simulink library "library"  (R2020a)
settings: Solver=VariableStepAuto  StartTime=0.0  StopTime=10.0  RelTol=1e-3
values from neighbouring files (symbols this model uses):
  height = 1080    [setup.m]    (also in setupSystem.m = heightName(nameIdx))
  nRho = maxRho*2    [setup.m]    (also in setupSystem.m)
  theta = (0:dTheta:180-dTheta)    [ARLHT.m]    (also in setup.m = (0:1:179); setupSystem.m = (0:1:179))
  width = 1920    [setup.m]    (also in setupSystem.m = widthName(nameIdx))
libraries: simulink x135, hdlsllib x83, $bdroot x15
(part 3 of 3)

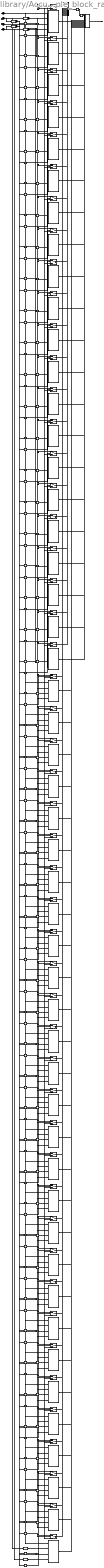
== system library/Accumulator Circuit/Accumulator Memory/Accumulator Memory/simple_block_ram ==
  wr_data : Inport
  wr_addr : Inport  Port=2
  wr_en : Inport  Port=3
  rd_addr : Inport  Port=4
  and_{0..48} (49 alike) : Logic  AllPortsSameDT=off  OutDataTypeStr=boolean
  bitwise_or : simulink/Logic and Bit Operations/Bitwise Operator  logicop=OR  UseBitMask=off  BitMask=bin2dec('11011001')  BitMaskRealWorld=Stored Integer
  constant_0 : Constant  Value=0  OutDataTypeStr=fixdt(0, 49, 0)  SampleTime=-1
  constant_1 : Constant  OutDataTypeStr=fixdt(0, 49, 0)  SampleTime=-1
  constant_10 : Constant  Value=10  OutDataTypeStr=fixdt(0, 49, 0)  SampleTime=-1
  constant_11 : Constant  Value=11  OutDataTypeStr=fixdt(0, 49, 0)  SampleTime=-1
  constant_12 : Constant  Value=12  OutDataTypeStr=fixdt(0, 49, 0)  SampleTime=-1
  constant_13 : Constant  Value=13  OutDataTypeStr=fixdt(0, 49, 0)  SampleTime=-1
  constant_14 : Constant  Value=14  OutDataTypeStr=fixdt(0, 49, 0)  SampleTime=-1
  constant_15 : Constant  Value=15  OutDataTypeStr=fixdt(0, 49, 0)  SampleTime=-1
  constant_16 : Constant  Value=16  OutDataTypeStr=fixdt(0, 49, 0)  SampleTime=-1
  constant_17 : Constant  Value=17  OutDataTypeStr=fixdt(0, 49, 0)  SampleTime=-1
  constant_18 : Constant  Value=18  OutDataTypeStr=fixdt(0, 49, 0)  SampleTime=-1
  constant_19 : Constant  Value=19  OutDataTypeStr=fixdt(0, 49, 0)  SampleTime=-1
  constant_2 : Constant  Value=2  OutDataTypeStr=fixdt(0, 49, 0)  SampleTime=-1
  constant_20 : Constant  Value=20  OutDataTypeStr=fixdt(0, 49, 0)  SampleTime=-1
  constant_21 : Constant  Value=21  OutDataTypeStr=fixdt(0, 49, 0)  SampleTime=-1
  constant_22 : Constant  Value=22  OutDataTypeStr=fixdt(0, 49, 0)  SampleTime=-1
  constant_23 : Constant  Value=23  OutDataTypeStr=fixdt(0, 49, 0)  SampleTime=-1
  constant_24 : Constant  Value=24  OutDataTypeStr=fixdt(0, 49, 0)  SampleTime=-1
  constant_25 : Constant  Value=25  OutDataTypeStr=fixdt(0, 49, 0)  SampleTime=-1
  constant_26 : Constant  Value=26  OutDataTypeStr=fixdt(0, 49, 0)  SampleTime=-1
  constant_27 : Constant  Value=27  OutDataTypeStr=fixdt(0, 49, 0)  SampleTime=-1
  constant_28 : Constant  Value=28  OutDataTypeStr=fixdt(0, 49, 0)  SampleTime=-1
  constant_29 : Constant  Value=29  OutDataTypeStr=fixdt(0, 49, 0)  SampleTime=-1
  constant_3 : Constant  Value=3  OutDataTypeStr=fixdt(0, 49, 0)  SampleTime=-1
  constant_30 : Constant  Value=30  OutDataTypeStr=fixdt(0, 49, 0)  SampleTime=-1
  constant_31 : Constant  Value=31  OutDataTypeStr=fixdt(0, 49, 0)  SampleTime=-1
  constant_32 : Constant  Value=32  OutDataTypeStr=fixdt(0, 49, 0)  SampleTime=-1
  constant_33 : Constant  Value=33  OutDataTypeStr=fixdt(0, 49, 0)  SampleTime=-1
  constant_34 : Constant  Value=34  OutDataTypeStr=fixdt(0, 49, 0)  SampleTime=-1
  constant_35 : Constant  Value=35  OutDataTypeStr=fixdt(0, 49, 0)  SampleTime=-1
  constant_36 : Constant  Value=36  OutDataTypeStr=fixdt(0, 49, 0)  SampleTime=-1
  constant_37 : Constant  Value=37  OutDataTypeStr=fixdt(0, 49, 0)  SampleTime=-1
  constant_38 : Constant  Value=38  OutDataTypeStr=fixdt(0, 49, 0)  SampleTime=-1
  constant_39 : Constant  Value=39  OutDataTypeStr=fixdt(0, 49, 0)  SampleTime=-1
  constant_4 : Constant  Value=4  OutDataTypeStr=fixdt(0, 49, 0)  SampleTime=-1
  constant_40 : Constant  Value=40  OutDataTypeStr=fixdt(0, 49, 0)  SampleTime=-1
  constant_41 : Constant  Value=41  OutDataTypeStr=fixdt(0, 49, 0)  SampleTime=-1
  constant_42 : Constant  Value=42  OutDataTypeStr=fixdt(0, 49, 0)  SampleTime=-1
  constant_43 : Constant  Value=43  OutDataTypeStr=fixdt(0, 49, 0)  SampleTime=-1
  constant_44 : Constant  Value=44  OutDataTypeStr=fixdt(0, 49, 0)  SampleTime=-1
  constant_45 : Constant  Value=45  OutDataTypeStr=fixdt(0, 49, 0)  SampleTime=-1
  constant_46 : Constant  Value=46  OutDataTypeStr=fixdt(0, 49, 0)  SampleTime=-1
  constant_47 : Constant  Value=47  OutDataTypeStr=fixdt(0, 49, 0)  SampleTime=-1
  constant_48 : Constant  Value=48  OutDataTypeStr=fixdt(0, 49, 0)  SampleTime=-1
  constant_5 : Constant  Value=5  OutDataTypeStr=fixdt(0, 49, 0)  SampleTime=-1
  constant_6 : Constant  Value=6  OutDataTypeStr=fixdt(0, 49, 0)  SampleTime=-1
  constant_7 : Constant  Value=7  OutDataTypeStr=fixdt(0, 49, 0)  SampleTime=-1
  constant_8 : Constant  Value=8  OutDataTypeStr=fixdt(0, 49, 0)  SampleTime=-1
  constant_9 : Constant  Value=9  OutDataTypeStr=fixdt(0, 49, 0)  SampleTime=-1
  delay : Delay  DelayLength=1
  multiport_switch : MultiPortSwitch  DataPortOrder=Zero-based contiguous  Inputs=49  zeroidx=on
  rd_address : hdlsllib/Logic and Bit Operations/Bit Slice  lidx=10  ridx=0
      settings: SourceProductBaseCode=SL
  rd_address_hr : hdlsllib/Logic and Bit Operations/Bit Slice  lidx=9  ridx=0
      settings: SourceProductBaseCode=SL
  rd_bitslice : hdlsllib/Logic and Bit Operations/Bit Slice  lidx=16  ridx=11
      settings: SourceProductBaseCode=SL
  rd_cmp2const_0 : simulink/Logic and Bit Operations/Compare To Constant  relop===  const=0  OutDataTypeStr=boolean
  rd_cmp2const_1 : simulink/Logic and Bit Operations/Compare To Constant  relop===  const=1  OutDataTypeStr=boolean
  rd_cmp2const_10 : simulink/Logic and Bit Operations/Compare To Constant  relop===  const=10  OutDataTypeStr=boolean
  rd_cmp2const_11 : simulink/Logic and Bit Operations/Compare To Constant  relop===  const=11  OutDataTypeStr=boolean
  rd_cmp2const_12 : simulink/Logic and Bit Operations/Compare To Constant  relop===  const=12  OutDataTypeStr=boolean
  rd_cmp2const_13 : simulink/Logic and Bit Operations/Compare To Constant  relop===  const=13  OutDataTypeStr=boolean
  rd_cmp2const_14 : simulink/Logic and Bit Operations/Compare To Constant  relop===  const=14  OutDataTypeStr=boolean
  rd_cmp2const_15 : simulink/Logic and Bit Operations/Compare To Constant  relop===  const=15  OutDataTypeStr=boolean
  rd_cmp2const_16 : simulink/Logic and Bit Operations/Compare To Constant  relop===  const=16  OutDataTypeStr=boolean
  rd_cmp2const_17 : simulink/Logic and Bit Operations/Compare To Constant  relop===  const=17  OutDataTypeStr=boolean
  rd_cmp2const_18 : simulink/Logic and Bit Operations/Compare To Constant  relop===  const=18  OutDataTypeStr=boolean
  rd_cmp2const_19 : simulink/Logic and Bit Operations/Compare To Constant  relop===  const=19  OutDataTypeStr=boolean
  rd_cmp2const_2 : simulink/Logic and Bit Operations/Compare To Constant  relop===  const=2  OutDataTypeStr=boolean
  rd_cmp2const_20 : simulink/Logic and Bit Operations/Compare To Constant  relop===  const=20  OutDataTypeStr=boolean
  rd_cmp2const_21 : simulink/Logic and Bit Operations/Compare To Constant  relop===  const=21  OutDataTypeStr=boolean
  rd_cmp2const_22 : simulink/Logic and Bit Operations/Compare To Constant  relop===  const=22  OutDataTypeStr=boolean
  rd_cmp2const_23 : simulink/Logic and Bit Operations/Compare To Constant  relop===  const=23  OutDataTypeStr=boolean
  rd_cmp2const_24 : simulink/Logic and Bit Operations/Compare To Constant  relop===  const=24  OutDataTypeStr=boolean
  rd_cmp2const_25 : simulink/Logic and Bit Operations/Compare To Constant  relop===  const=25  OutDataTypeStr=boolean
  rd_cmp2const_26 : simulink/Logic and Bit Operations/Compare To Constant  relop===  const=26  OutDataTypeStr=boolean
  rd_cmp2const_27 : simulink/Logic and Bit Operations/Compare To Constant  relop===  const=27  OutDataTypeStr=boolean
  rd_cmp2const_28 : simulink/Logic and Bit Operations/Compare To Constant  relop===  const=28  OutDataTypeStr=boolean
  rd_cmp2const_29 : simulink/Logic and Bit Operations/Compare To Constant  relop===  const=29  OutDataTypeStr=boolean
  rd_cmp2const_3 : simulink/Logic and Bit Operations/Compare To Constant  relop===  const=3  OutDataTypeStr=boolean
  rd_cmp2const_30 : simulink/Logic and Bit Operations/Compare To Constant  relop===  const=30  OutDataTypeStr=boolean
  rd_cmp2const_31 : simulink/Logic and Bit Operations/Compare To Constant  relop===  const=31  OutDataTypeStr=boolean
  rd_cmp2const_32 : simulink/Logic and Bit Operations/Compare To Constant  relop===  const=32  OutDataTypeStr=boolean
  rd_cmp2const_33 : simulink/Logic and Bit Operations/Compare To Constant  relop===  const=33  OutDataTypeStr=boolean
  rd_cmp2const_34 : simulink/Logic and Bit Operations/Compare To Constant  relop===  const=34  OutDataTypeStr=boolean
  rd_cmp2const_35 : simulink/Logic and Bit Operations/Compare To Constant  relop===  const=35  OutDataTypeStr=boolean
  rd_cmp2const_36 : simulink/Logic and Bit Operations/Compare To Constant  relop===  const=36  OutDataTypeStr=boolean
  rd_cmp2const_37 : simulink/Logic and Bit Operations/Compare To Constant  relop===  const=37  OutDataTypeStr=boolean
  rd_cmp2const_38 : simulink/Logic and Bit Operations/Compare To Constant  relop===  const=38  OutDataTypeStr=boolean
  rd_cmp2const_39 : simulink/Logic and Bit Operations/Compare To Constant  relop===  const=39  OutDataTypeStr=boolean
  rd_cmp2const_4 : simulink/Logic and Bit Operations/Compare To Constant  relop===  const=4  OutDataTypeStr=boolean
  rd_cmp2const_40 : simulink/Logic and Bit Operations/Compare To Constant  relop===  const=40  OutDataTypeStr=boolean
  rd_cmp2const_41 : simulink/Logic and Bit Operations/Compare To Constant  relop===  const=41  OutDataTypeStr=boolean
  rd_cmp2const_42 : simulink/Logic and Bit Operations/Compare To Constant  relop===  const=42  OutDataTypeStr=boolean
  rd_cmp2const_43 : simulink/Logic and Bit Operations/Compare To Constant  relop===  const=43  OutDataTypeStr=boolean
  rd_cmp2const_44 : simulink/Logic and Bit Operations/Compare To Constant  relop===  const=44  OutDataTypeStr=boolean
  rd_cmp2const_45 : simulink/Logic and Bit Operations/Compare To Constant  relop===  const=45  OutDataTypeStr=boolean
  rd_cmp2const_46 : simulink/Logic and Bit Operations/Compare To Constant  relop===  const=46  OutDataTypeStr=boolean
  rd_cmp2const_47 : simulink/Logic and Bit Operations/Compare To Constant  relop===  const=47  OutDataTypeStr=boolean
  rd_cmp2const_48 : simulink/Logic and Bit Operations/Compare To Constant  relop===  const=48  OutDataTypeStr=boolean
  rd_cmp2const_5 : simulink/Logic and Bit Operations/Compare To Constant  relop===  const=5  OutDataTypeStr=boolean
  rd_cmp2const_6 : simulink/Logic and Bit Operations/Compare To Constant  relop===  const=6  OutDataTypeStr=boolean
  rd_cmp2const_7 : simulink/Logic and Bit Operations/Compare To Constant  relop===  const=7  OutDataTypeStr=boolean
  rd_cmp2const_8 : simulink/Logic and Bit Operations/Compare To Constant  relop===  const=8  OutDataTypeStr=boolean
  rd_cmp2const_9 : simulink/Logic and Bit Operations/Compare To Constant  relop===  const=9  OutDataTypeStr=boolean
  simple_ram_{0..47} (48 alike) : hdlsllib/HDL RAMs/Simple Dual Port RAM  ram_size=11
      settings: SourceProductBaseCode=SL
  simple_ram_48 : hdlsllib/HDL RAMs/Simple Dual Port RAM  ram_size=10
      settings: SourceProductBaseCode=SL
  switch_{0..48} (49 alike) : Switch  Threshold=1
  vector_concatenate : Concatenate  NumInputs=49
  wr_address : hdlsllib/Logic and Bit Operations/Bit Slice  lidx=10  ridx=0
      settings: SourceProductBaseCode=SL
  wr_address_hr : hdlsllib/Logic and Bit Operations/Bit Slice  lidx=9  ridx=0
      settings: SourceProductBaseCode=SL
  wr_bitslice : hdlsllib/Logic and Bit Operations/Bit Slice  lidx=16  ridx=11
      settings: SourceProductBaseCode=SL
  wr_cmp2const_0 : simulink/Logic and Bit Operations/Compare To Constant  relop===  const=0  OutDataTypeStr=boolean
  wr_cmp2const_1 : simulink/Logic and Bit Operations/Compare To Constant  relop===  const=1  OutDataTypeStr=boolean
  wr_cmp2const_10 : simulink/Logic and Bit Operations/Compare To Constant  relop===  const=10  OutDataTypeStr=boolean
  wr_cmp2const_11 : simulink/Logic and Bit Operations/Compare To Constant  relop===  const=11  OutDataTypeStr=boolean
  wr_cmp2const_12 : simulink/Logic and Bit Operations/Compare To Constant  relop===  const=12  OutDataTypeStr=boolean
  wr_cmp2const_13 : simulink/Logic and Bit Operations/Compare To Constant  relop===  const=13  OutDataTypeStr=boolean
  wr_cmp2const_14 : simulink/Logic and Bit Operations/Compare To Constant  relop===  const=14  OutDataTypeStr=boolean
  wr_cmp2const_15 : simulink/Logic and Bit Operations/Compare To Constant  relop===  const=15  OutDataTypeStr=boolean
  wr_cmp2const_16 : simulink/Logic and Bit Operations/Compare To Constant  relop===  const=16  OutDataTypeStr=boolean
  wr_cmp2const_17 : simulink/Logic and Bit Operations/Compare To Constant  relop===  const=17  OutDataTypeStr=boolean
  wr_cmp2const_18 : simulink/Logic and Bit Operations/Compare To Constant  relop===  const=18  OutDataTypeStr=boolean
  wr_cmp2const_19 : simulink/Logic and Bit Operations/Compare To Constant  relop===  const=19  OutDataTypeStr=boolean
  wr_cmp2const_2 : simulink/Logic and Bit Operations/Compare To Constant  relop===  const=2  OutDataTypeStr=boolean
  wr_cmp2const_20 : simulink/Logic and Bit Operations/Compare To Constant  relop===  const=20  OutDataTypeStr=boolean
  wr_cmp2const_21 : simulink/Logic and Bit Operations/Compare To Constant  relop===  const=21  OutDataTypeStr=boolean
  wr_cmp2const_22 : simulink/Logic and Bit Operations/Compare To Constant  relop===  const=22  OutDataTypeStr=boolean
  wr_cmp2const_23 : simulink/Logic and Bit Operations/Compare To Constant  relop===  const=23  OutDataTypeStr=boolean
  wr_cmp2const_24 : simulink/Logic and Bit Operations/Compare To Constant  relop===  const=24  OutDataTypeStr=boolean
  wr_cmp2const_25 : simulink/Logic and Bit Operations/Compare To Constant  relop===  const=25  OutDataTypeStr=boolean
  wr_cmp2const_26 : simulink/Logic and Bit Operations/Compare To Constant  relop===  const=26  OutDataTypeStr=boolean
  wr_cmp2const_27 : simulink/Logic and Bit Operations/Compare To Constant  relop===  const=27  OutDataTypeStr=boolean
  wr_cmp2const_28 : simulink/Logic and Bit Operations/Compare To Constant  relop===  const=28  OutDataTypeStr=boolean
  wr_cmp2const_29 : simulink/Logic and Bit Operations/Compare To Constant  relop===  const=29  OutDataTypeStr=boolean
  wr_cmp2const_3 : simulink/Logic and Bit Operations/Compare To Constant  relop===  const=3  OutDataTypeStr=boolean
  wr_cmp2const_30 : simulink/Logic and Bit Operations/Compare To Constant  relop===  const=30  OutDataTypeStr=boolean
  wr_cmp2const_31 : simulink/Logic and Bit Operations/Compare To Constant  relop===  const=31  OutDataTypeStr=boolean
  wr_cmp2const_32 : simulink/Logic and Bit Operations/Compare To Constant  relop===  const=32  OutDataTypeStr=boolean
  wr_cmp2const_33 : simulink/Logic and Bit Operations/Compare To Constant  relop===  const=33  OutDataTypeStr=boolean
  wr_cmp2const_34 : simulink/Logic and Bit Operations/Compare To Constant  relop===  const=34  OutDataTypeStr=boolean
  wr_cmp2const_35 : simulink/Logic and Bit Operations/Compare To Constant  relop===  const=35  OutDataTypeStr=boolean
  wr_cmp2const_36 : simulink/Logic and Bit Operations/Compare To Constant  relop===  const=36  OutDataTypeStr=boolean
  wr_cmp2const_37 : simulink/Logic and Bit Operations/Compare To Constant  relop===  const=37  OutDataTypeStr=boolean
  wr_cmp2const_38 : simulink/Logic and Bit Operations/Compare To Constant  relop===  const=38  OutDataTypeStr=boolean
  wr_cmp2const_39 : simulink/Logic and Bit Operations/Compare To Constant  relop===  const=39  OutDataTypeStr=boolean
  wr_cmp2const_4 : simulink/Logic and Bit Operations/Compare To Constant  relop===  const=4  OutDataTypeStr=boolean
  wr_cmp2const_40 : simulink/Logic and Bit Operations/Compare To Constant  relop===  const=40  OutDataTypeStr=boolean
  wr_cmp2const_41 : simulink/Logic and Bit Operations/Compare To Constant  relop===  const=41  OutDataTypeStr=boolean
  wr_cmp2const_42 : simulink/Logic and Bit Operations/Compare To Constant  relop===  const=42  OutDataTypeStr=boolean
  wr_cmp2const_43 : simulink/Logic and Bit Operations/Compare To Constant  relop===  const=43  OutDataTypeStr=boolean
  wr_cmp2const_44 : simulink/Logic and Bit Operations/Compare To Constant  relop===  const=44  OutDataTypeStr=boolean
  wr_cmp2const_45 : simulink/Logic and Bit Operations/Compare To Constant  relop===  const=45  OutDataTypeStr=boolean
  wr_cmp2const_46 : simulink/Logic and Bit Operations/Compare To Constant  relop===  const=46  OutDataTypeStr=boolean
  wr_cmp2const_47 : simulink/Logic and Bit Operations/Compare To Constant  relop===  const=47  OutDataTypeStr=boolean
  wr_cmp2const_48 : simulink/Logic and Bit Operations/Compare To Constant  relop===  const=48  OutDataTypeStr=boolean
  wr_cmp2const_5 : simulink/Logic and Bit Operations/Compare To Constant  relop===  const=5  OutDataTypeStr=boolean
  wr_cmp2const_6 : simulink/Logic and Bit Operations/Compare To Constant  relop===  const=6  OutDataTypeStr=boolean
  wr_cmp2const_7 : simulink/Logic and Bit Operations/Compare To Constant  relop===  const=7  OutDataTypeStr=boolean
  wr_cmp2const_8 : simulink/Logic and Bit Operations/Compare To Constant  relop===  const=8  OutDataTypeStr=boolean
  wr_cmp2const_9 : simulink/Logic and Bit Operations/Compare To Constant  relop===  const=9  OutDataTypeStr=boolean
  zero : Constant  Value=0  OutDataTypeStr=fixdt(0, 49, 0)  SampleTime=-1
  rd_data : Outport
  wires:
  wr_data/1 -> simple_ram_0/1, simple_ram_1/1, simple_ram_2/1, simple_ram_3/1, simple_ram_4/1, simple_ram_5/1, simple_ram_6/1, simple_ram_7/1, simple_ram_8/1, simple_ram_9/1, simple_ram_10/1, simple_ram_11/1, simple_ram_12/1, simple_ram_13/1, simple_ram_14/1, simple_ram_15/1, simple_ram_16/1, simple_ram_17/1, simple_ram_18/1, simple_ram_19/1, simple_ram_20/1, simple_ram_21/1, simple_ram_22/1, simple_ram_23/1, simple_ram_24/1, simple_ram_25/1, simple_ram_26/1, simple_ram_27/1, simple_ram_28/1, simple_ram_29/1, simple_ram_30/1, simple_ram_31/1, simple_ram_32/1, simple_ram_33/1, simple_ram_34/1, simple_ram_35/1, simple_ram_36/1, simple_ram_37/1, simple_ram_38/1, simple_ram_39/1, simple_ram_40/1, simple_ram_41/1, simple_ram_42/1, simple_ram_43/1, simple_ram_44/1, simple_ram_45/1, simple_ram_46/1, simple_ram_47/1, simple_ram_48/1
  wr_address/1 -> simple_ram_0/2, simple_ram_1/2, simple_ram_2/2, simple_ram_3/2, simple_ram_4/2, simple_ram_5/2, simple_ram_6/2, simple_ram_7/2, simple_ram_8/2, simple_ram_9/2, simple_ram_10/2, simple_ram_11/2, simple_ram_12/2, simple_ram_13/2, simple_ram_14/2, simple_ram_15/2, simple_ram_16/2, simple_ram_17/2, simple_ram_18/2, simple_ram_19/2, simple_ram_20/2, simple_ram_21/2, simple_ram_22/2, simple_ram_23/2, simple_ram_24/2, simple_ram_25/2, simple_ram_26/2, simple_ram_27/2, simple_ram_28/2, simple_ram_29/2, simple_ram_30/2, simple_ram_31/2, simple_ram_32/2, simple_ram_33/2, simple_ram_34/2, simple_ram_35/2, simple_ram_36/2, simple_ram_37/2, simple_ram_38/2, simple_ram_39/2, simple_ram_40/2, simple_ram_41/2, simple_ram_42/2, simple_ram_43/2, simple_ram_44/2, simple_ram_45/2, simple_ram_46/2, simple_ram_47/2
  rd_address/1 -> simple_ram_0/4, simple_ram_1/4, simple_ram_2/4, simple_ram_3/4, simple_ram_4/4, simple_ram_5/4, simple_ram_6/4, simple_ram_7/4, simple_ram_8/4, simple_ram_9/4, simple_ram_10/4, simple_ram_11/4, simple_ram_12/4, simple_ram_13/4, simple_ram_14/4, simple_ram_15/4, simple_ram_16/4, simple_ram_17/4, simple_ram_18/4, simple_ram_19/4, simple_ram_20/4, simple_ram_21/4, simple_ram_22/4, simple_ram_23/4, simple_ram_24/4, simple_ram_25/4, simple_ram_26/4, simple_ram_27/4, simple_ram_28/4, simple_ram_29/4, simple_ram_30/4, simple_ram_31/4, simple_ram_32/4, simple_ram_33/4, simple_ram_34/4, simple_ram_35/4, simple_ram_36/4, simple_ram_37/4, simple_ram_38/4, simple_ram_39/4, simple_ram_40/4, simple_ram_41/4, simple_ram_42/4, simple_ram_43/4, simple_ram_44/4, simple_ram_45/4, simple_ram_46/4, simple_ram_47/4
  constant_0/1 -> switch_0/1
  zero/1 -> switch_0/3, switch_1/3, switch_2/3, switch_3/3, switch_4/3, switch_5/3, switch_6/3, switch_7/3, switch_8/3, switch_9/3, switch_10/3, switch_11/3, switch_12/3, switch_13/3, switch_14/3, switch_15/3, switch_16/3, switch_17/3, switch_18/3, switch_19/3, switch_20/3, switch_21/3, switch_22/3, switch_23/3, switch_24/3, switch_25/3, switch_26/3, switch_27/3, switch_28/3, switch_29/3, switch_30/3, switch_31/3, switch_32/3, switch_33/3, switch_34/3, switch_35/3, switch_36/3, switch_37/3, switch_38/3, switch_39/3, switch_40/3, switch_41/3, switch_42/3, switch_43/3, switch_44/3, switch_45/3, switch_46/3, switch_47/3, switch_48/3
  switch_0/1 -> vector_concatenate/1
  simple_ram_0/1 -> multiport_switch/2
  wr_bitslice/1 -> wr_cmp2const_0/1, wr_cmp2const_1/1, wr_cmp2const_2/1, wr_cmp2const_3/1, wr_cmp2const_4/1, wr_cmp2const_5/1, wr_cmp2const_6/1, wr_cmp2const_7/1, wr_cmp2const_8/1, wr_cmp2const_9/1, wr_cmp2const_10/1, wr_cmp2const_11/1, wr_cmp2const_12/1, wr_cmp2const_13/1, wr_cmp2const_14/1, wr_cmp2const_15/1, wr_cmp2const_16/1, wr_cmp2const_17/1, wr_cmp2const_18/1, wr_cmp2const_19/1, wr_cmp2const_20/1, wr_cmp2const_21/1, wr_cmp2const_22/1, wr_cmp2const_23/1, wr_cmp2const_24/1, wr_cmp2const_25/1, wr_cmp2const_26/1, wr_cmp2const_27/1, wr_cmp2const_28/1, wr_cmp2const_29/1, wr_cmp2const_30/1, wr_cmp2const_31/1, wr_cmp2const_32/1, wr_cmp2const_33/1, wr_cmp2const_34/1, wr_cmp2const_35/1, wr_cmp2const_36/1, wr_cmp2const_37/1, wr_cmp2const_38/1, wr_cmp2const_39/1, wr_cmp2const_40/1, wr_cmp2const_41/1, wr_cmp2const_42/1, wr_cmp2const_43/1, wr_cmp2const_44/1, wr_cmp2const_45/1, wr_cmp2const_46/1, wr_cmp2const_47/1, wr_cmp2const_48/1
  rd_bitslice/1 -> rd_cmp2const_0/1, rd_cmp2const_1/1, rd_cmp2const_2/1, rd_cmp2const_3/1, rd_cmp2const_4/1, rd_cmp2const_5/1, rd_cmp2const_6/1, rd_cmp2const_7/1, rd_cmp2const_8/1, rd_cmp2const_9/1, rd_cmp2const_10/1, rd_cmp2const_11/1, rd_cmp2const_12/1, rd_cmp2const_13/1, rd_cmp2const_14/1, rd_cmp2const_15/1, rd_cmp2const_16/1, rd_cmp2const_17/1, rd_cmp2const_18/1, rd_cmp2const_19/1, rd_cmp2const_20/1, rd_cmp2const_21/1, rd_cmp2const_22/1, rd_cmp2const_23/1, rd_cmp2const_24/1, rd_cmp2const_25/1, rd_cmp2const_26/1, rd_cmp2const_27/1, rd_cmp2const_28/1, rd_cmp2const_29/1, rd_cmp2const_30/1, rd_cmp2const_31/1, rd_cmp2const_32/1, rd_cmp2const_33/1, rd_cmp2const_34/1, rd_cmp2const_35/1, rd_cmp2const_36/1, rd_cmp2const_37/1, rd_cmp2const_38/1, rd_cmp2const_39/1, rd_cmp2const_40/1, rd_cmp2const_41/1, rd_cmp2const_42/1, rd_cmp2const_43/1, rd_cmp2const_44/1, rd_cmp2const_45/1, rd_cmp2const_46/1, rd_cmp2const_47/1, rd_cmp2const_48/1
  wr_en/1 -> and_0/2, and_1/2, and_2/2, and_3/2, and_4/2, and_5/2, and_6/2, and_7/2, and_8/2, and_9/2, and_10/2, and_11/2, and_12/2, and_13/2, and_14/2, and_15/2, and_16/2, and_17/2, and_18/2, and_19/2, and_20/2, and_21/2, and_22/2, and_23/2, and_24/2, and_25/2, and_26/2, and_27/2, and_28/2, and_29/2, and_30/2, and_31/2, and_32/2, and_33/2, and_34/2, and_35/2, and_36/2, and_37/2, and_38/2, and_39/2, and_40/2, and_41/2, and_42/2, and_43/2, and_44/2, and_45/2, and_46/2, and_47/2, and_48/2
  and_0/1 -> simple_ram_0/3
  wr_cmp2const_0/1 -> and_0/1
  rd_cmp2const_0/1 -> switch_0/2
  constant_1/1 -> switch_1/1
  switch_1/1 -> vector_concatenate/2
  simple_ram_1/1 -> multiport_switch/3
  and_1/1 -> simple_ram_1/3
  wr_cmp2const_1/1 -> and_1/1
  rd_cmp2const_1/1 -> switch_1/2
  constant_2/1 -> switch_2/1
  switch_2/1 -> vector_concatenate/3
  simple_ram_2/1 -> multiport_switch/4
  and_2/1 -> simple_ram_2/3
  wr_cmp2const_2/1 -> and_2/1
  rd_cmp2const_2/1 -> switch_2/2
  constant_3/1 -> switch_3/1
  switch_3/1 -> vector_concatenate/4
  simple_ram_3/1 -> multiport_switch/5
  and_3/1 -> simple_ram_3/3
  wr_cmp2const_3/1 -> and_3/1
  rd_cmp2const_3/1 -> switch_3/2
  constant_4/1 -> switch_4/1
  switch_4/1 -> vector_concatenate/5
  simple_ram_4/1 -> multiport_switch/6
  and_4/1 -> simple_ram_4/3
  wr_cmp2const_4/1 -> and_4/1
  rd_cmp2const_4/1 -> switch_4/2
  constant_5/1 -> switch_5/1
  switch_5/1 -> vector_concatenate/6
  simple_ram_5/1 -> multiport_switch/7
  and_5/1 -> simple_ram_5/3
  wr_cmp2const_5/1 -> and_5/1
  rd_cmp2const_5/1 -> switch_5/2
  constant_6/1 -> switch_6/1
  switch_6/1 -> vector_concatenate/7
  simple_ram_6/1 -> multiport_switch/8
  and_6/1 -> simple_ram_6/3
  wr_cmp2const_6/1 -> and_6/1
  rd_cmp2const_6/1 -> switch_6/2
  constant_7/1 -> switch_7/1
  switch_7/1 -> vector_concatenate/8
  simple_ram_7/1 -> multiport_switch/9
  and_7/1 -> simple_ram_7/3
  wr_cmp2const_7/1 -> and_7/1
  rd_cmp2const_7/1 -> switch_7/2
  constant_8/1 -> switch_8/1
  switch_8/1 -> vector_concatenate/9
  simple_ram_8/1 -> multiport_switch/10
  and_8/1 -> simple_ram_8/3
  wr_cmp2const_8/1 -> and_8/1
  rd_cmp2const_8/1 -> switch_8/2
  constant_9/1 -> switch_9/1
  switch_9/1 -> vector_concatenate/10
  simple_ram_9/1 -> multiport_switch/11
  and_9/1 -> simple_ram_9/3
  wr_cmp2const_9/1 -> and_9/1
  rd_cmp2const_9/1 -> switch_9/2
  constant_10/1 -> switch_10/1
  switch_10/1 -> vector_concatenate/11
  simple_ram_10/1 -> multiport_switch/12
  and_10/1 -> simple_ram_10/3
  wr_cmp2const_10/1 -> and_10/1
  rd_cmp2const_10/1 -> switch_10/2
  constant_11/1 -> switch_11/1
  switch_11/1 -> vector_concatenate/12
  simple_ram_11/1 -> multiport_switch/13
  and_11/1 -> simple_ram_11/3
  wr_cmp2const_11/1 -> and_11/1
  rd_cmp2const_11/1 -> switch_11/2
  constant_12/1 -> switch_12/1
  switch_12/1 -> vector_concatenate/13
  simple_ram_12/1 -> multiport_switch/14
  and_12/1 -> simple_ram_12/3
  wr_cmp2const_12/1 -> and_12/1
  rd_cmp2const_12/1 -> switch_12/2
  constant_13/1 -> switch_13/1
  switch_13/1 -> vector_concatenate/14
  simple_ram_13/1 -> multiport_switch/15
  and_13/1 -> simple_ram_13/3
  wr_cmp2const_13/1 -> and_13/1
  rd_cmp2const_13/1 -> switch_13/2
  constant_14/1 -> switch_14/1
  switch_14/1 -> vector_concatenate/15
  simple_ram_14/1 -> multiport_switch/16
  and_14/1 -> simple_ram_14/3
  wr_cmp2const_14/1 -> and_14/1
  rd_cmp2const_14/1 -> switch_14/2
  constant_15/1 -> switch_15/1
  switch_15/1 -> vector_concatenate/16
  simple_ram_15/1 -> multiport_switch/17
  and_15/1 -> simple_ram_15/3
  wr_cmp2const_15/1 -> and_15/1
  rd_cmp2const_15/1 -> switch_15/2
  constant_16/1 -> switch_16/1
  switch_16/1 -> vector_concatenate/17
  simple_ram_16/1 -> multiport_switch/18
  and_16/1 -> simple_ram_16/3
  wr_cmp2const_16/1 -> and_16/1
  rd_cmp2const_16/1 -> switch_16/2
  constant_17/1 -> switch_17/1
  switch_17/1 -> vector_concatenate/18
  simple_ram_17/1 -> multiport_switch/19
  and_17/1 -> simple_ram_17/3
  wr_cmp2const_17/1 -> and_17/1
  rd_cmp2const_17/1 -> switch_17/2
  constant_18/1 -> switch_18/1
  switch_18/1 -> vector_concatenate/19
  simple_ram_18/1 -> multiport_switch/20
  and_18/1 -> simple_ram_18/3
  wr_cmp2const_18/1 -> and_18/1
  rd_cmp2const_18/1 -> switch_18/2
  constant_19/1 -> switch_19/1
  switch_19/1 -> vector_concatenate/20
  simple_ram_19/1 -> multiport_switch/21
  and_19/1 -> simple_ram_19/3
  wr_cmp2const_19/1 -> and_19/1
  rd_cmp2const_19/1 -> switch_19/2
  constant_20/1 -> switch_20/1
  switch_20/1 -> vector_concatenate/21
  simple_ram_20/1 -> multiport_switch/22
  and_20/1 -> simple_ram_20/3
  wr_cmp2const_20/1 -> and_20/1
  rd_cmp2const_20/1 -> switch_20/2
  constant_21/1 -> switch_21/1
  switch_21/1 -> vector_concatenate/22
  simple_ram_21/1 -> multiport_switch/23
  and_21/1 -> simple_ram_21/3
  wr_cmp2const_21/1 -> and_21/1
  rd_cmp2const_21/1 -> switch_21/2
  constant_22/1 -> switch_22/1
  switch_22/1 -> vector_concatenate/23
  simple_ram_22/1 -> multiport_switch/24
  and_22/1 -> simple_ram_22/3
  wr_cmp2const_22/1 -> and_22/1
  rd_cmp2const_22/1 -> switch_22/2
  constant_23/1 -> switch_23/1
  switch_23/1 -> vector_concatenate/24
  simple_ram_23/1 -> multiport_switch/25
  and_23/1 -> simple_ram_23/3
  wr_cmp2const_23/1 -> and_23/1
  rd_cmp2const_23/1 -> switch_23/2
  constant_24/1 -> switch_24/1
  switch_24/1 -> vector_concatenate/25
  simple_ram_24/1 -> multiport_switch/26
  and_24/1 -> simple_ram_24/3
  wr_cmp2const_24/1 -> and_24/1
  rd_cmp2const_24/1 -> switch_24/2
  constant_25/1 -> switch_25/1
  switch_25/1 -> vector_concatenate/26
  simple_ram_25/1 -> multiport_switch/27
  and_25/1 -> simple_ram_25/3
  wr_cmp2const_25/1 -> and_25/1
  rd_cmp2const_25/1 -> switch_25/2
  constant_26/1 -> switch_26/1
  switch_26/1 -> vector_concatenate/27
  simple_ram_26/1 -> multiport_switch/28
  and_26/1 -> simple_ram_26/3
  wr_cmp2const_26/1 -> and_26/1
  rd_cmp2const_26/1 -> switch_26/2
  constant_27/1 -> switch_27/1
  switch_27/1 -> vector_concatenate/28
  simple_ram_27/1 -> multiport_switch/29
  and_27/1 -> simple_ram_27/3
  wr_cmp2const_27/1 -> and_27/1
  rd_cmp2const_27/1 -> switch_27/2
  constant_28/1 -> switch_28/1
  switch_28/1 -> vector_concatenate/29
  simple_ram_28/1 -> multiport_switch/30
  and_28/1 -> simple_ram_28/3
  wr_cmp2const_28/1 -> and_28/1
  rd_cmp2const_28/1 -> switch_28/2
  constant_29/1 -> switch_29/1
  switch_29/1 -> vector_concatenate/30
  simple_ram_29/1 -> multiport_switch/31
  and_29/1 -> simple_ram_29/3
  wr_cmp2const_29/1 -> and_29/1
  rd_cmp2const_29/1 -> switch_29/2
  constant_30/1 -> switch_30/1
  switch_30/1 -> vector_concatenate/31
  simple_ram_30/1 -> multiport_switch/32
  and_30/1 -> simple_ram_30/3
  wr_cmp2const_30/1 -> and_30/1
  rd_cmp2const_30/1 -> switch_30/2
  constant_31/1 -> switch_31/1
  switch_31/1 -> vector_concatenate/32
  simple_ram_31/1 -> multiport_switch/33
  and_31/1 -> simple_ram_31/3
  wr_cmp2const_31/1 -> and_31/1
  rd_cmp2const_31/1 -> switch_31/2
  constant_32/1 -> switch_32/1
  switch_32/1 -> vector_concatenate/33
  simple_ram_32/1 -> multiport_switch/34
  and_32/1 -> simple_ram_32/3
  wr_cmp2const_32/1 -> and_32/1
  rd_cmp2const_32/1 -> switch_32/2
  constant_33/1 -> switch_33/1
  switch_33/1 -> vector_concatenate/34
  simple_ram_33/1 -> multiport_switch/35
  and_33/1 -> simple_ram_33/3
  wr_cmp2const_33/1 -> and_33/1
  rd_cmp2const_33/1 -> switch_33/2
  constant_34/1 -> switch_34/1
  switch_34/1 -> vector_concatenate/35
  simple_ram_34/1 -> multiport_switch/36
  and_34/1 -> simple_ram_34/3
  wr_cmp2const_34/1 -> and_34/1
  rd_cmp2const_34/1 -> switch_34/2
  constant_35/1 -> switch_35/1
  switch_35/1 -> vector_concatenate/36
  simple_ram_35/1 -> multiport_switch/37
  and_35/1 -> simple_ram_35/3
  wr_cmp2const_35/1 -> and_35/1
  rd_cmp2const_35/1 -> switch_35/2
  constant_36/1 -> switch_36/1
  switch_36/1 -> vector_concatenate/37
  simple_ram_36/1 -> multiport_switch/38
  and_36/1 -> simple_ram_36/3
  wr_cmp2const_36/1 -> and_36/1
  rd_cmp2const_36/1 -> switch_36/2
  constant_37/1 -> switch_37/1
  switch_37/1 -> vector_concatenate/38
  simple_ram_37/1 -> multiport_switch/39
  and_37/1 -> simple_ram_37/3
  wr_cmp2const_37/1 -> and_37/1
  rd_cmp2const_37/1 -> switch_37/2
  constant_38/1 -> switch_38/1
  switch_38/1 -> vector_concatenate/39
  simple_ram_38/1 -> multiport_switch/40
  and_38/1 -> simple_ram_38/3
  wr_cmp2const_38/1 -> and_38/1
  rd_cmp2const_38/1 -> switch_38/2
  constant_39/1 -> switch_39/1
  switch_39/1 -> vector_concatenate/40
  simple_ram_39/1 -> multiport_switch/41
  and_39/1 -> simple_ram_39/3
  wr_cmp2const_39/1 -> and_39/1
  rd_cmp2const_39/1 -> switch_39/2
  constant_40/1 -> switch_40/1
  switch_40/1 -> vector_concatenate/41
  simple_ram_40/1 -> multiport_switch/42
  and_40/1 -> simple_ram_40/3
  wr_cmp2const_40/1 -> and_40/1
  rd_cmp2const_40/1 -> switch_40/2
  constant_41/1 -> switch_41/1
  switch_41/1 -> vector_concatenate/42
  simple_ram_41/1 -> multiport_switch/43
  and_41/1 -> simple_ram_41/3
  wr_cmp2const_41/1 -> and_41/1
  rd_cmp2const_41/1 -> switch_41/2
  constant_42/1 -> switch_42/1
  switch_42/1 -> vector_concatenate/43
  simple_ram_42/1 -> multiport_switch/44
  and_42/1 -> simple_ram_42/3
  wr_cmp2const_42/1 -> and_42/1
  rd_cmp2const_42/1 -> switch_42/2
  constant_43/1 -> switch_43/1
  switch_43/1 -> vector_concatenate/44
  simple_ram_43/1 -> multiport_switch/45
  and_43/1 -> simple_ram_43/3
  wr_cmp2const_43/1 -> and_43/1
  rd_cmp2const_43/1 -> switch_43/2
  constant_44/1 -> switch_44/1
  switch_44/1 -> vector_concatenate/45
  simple_ram_44/1 -> multiport_switch/46
  and_44/1 -> simple_ram_44/3
  wr_cmp2const_44/1 -> and_44/1
  rd_cmp2const_44/1 -> switch_44/2
  constant_45/1 -> switch_45/1
  switch_45/1 -> vector_concatenate/46
  simple_ram_45/1 -> multiport_switch/47
  and_45/1 -> simple_ram_45/3
  wr_cmp2const_45/1 -> and_45/1
  rd_cmp2const_45/1 -> switch_45/2
  constant_46/1 -> switch_46/1
  switch_46/1 -> vector_concatenate/47
  simple_ram_46/1 -> multiport_switch/48
  and_46/1 -> simple_ram_46/3
  wr_cmp2const_46/1 -> and_46/1
  rd_cmp2const_46/1 -> switch_46/2
  constant_47/1 -> switch_47/1
  switch_47/1 -> vector_concatenate/48
  simple_ram_47/1 -> multiport_switch/49
  and_47/1 -> simple_ram_47/3
  wr_cmp2const_47/1 -> and_47/1
  rd_cmp2const_47/1 -> switch_47/2
  constant_48/1 -> switch_48/1
  switch_48/1 -> vector_concatenate/49
  simple_ram_48/1 -> multiport_switch/50
  and_48/1 -> simple_ram_48/3
  wr_cmp2const_48/1 -> and_48/1
  rd_cmp2const_48/1 -> switch_48/2
  rd_addr/1 -> rd_bitslice/1, rd_address/1, rd_address_hr/1
  wr_addr/1 -> wr_bitslice/1, wr_address/1, wr_address_hr/1
  vector_concatenate/1 -> bitwise_or/1
  bitwise_or/1 -> delay/1
  delay/1 -> multiport_switch/1
  multiport_switch/1 -> rd_data/1
  wr_address_hr/1 -> simple_ram_48/2
  rd_address_hr/1 -> simple_ram_48/4

== matlab function library/Accumulator Circuit/MATLAB Function ==
  data: sof input; mode output; rho_address output; theta_address output; eof input; ntheta input; nrho input; ktheta input; clear output; valid output; debug_state output
function [mode, rho_address, theta_address, clear, valid, debug_state] = fcn(sof, eof, ntheta, nrho, ktheta)

IDLE = fi(0, 0, 2, 0);
VOTE = fi(1, 0, 2, 0);
READ = fi(2, 0, 2, 0);
CLEAR = fi(3, 0, 2, 0);

persistent current_state;
persistent rho_count;
persistent theta_count;
persistent k_count;

if isempty(current_state)
    current_state = IDLE;
end

if isempty(rho_count)
    rho_count = fi(0, 0, 16, 0);
end

if isempty(theta_count)
    theta_count = fi(0, 0, 8, 0);
end

if isempty(k_count)
    k_count = fi(0, 0, 8, 0);
end

switch current_state
    case IDLE
        mode = false;
        valid = false;
        clear = false;
        rho_address = rho_count;
        theta_address = theta_count;
        debug_state = IDLE;
        
        if sof
            current_state = VOTE;
        else
            current_state = IDLE;
        end
        
    case VOTE
        mode = true;
        valid = false;
        clear = false;
        rho_address = rho_count;
        theta_address = theta_count;
        debug_state = VOTE;
        
        if eof
            current_state = READ;
        else
            current_state = VOTE;
        end
        
    case READ
        mode = false;
        valid = true;
        clear = false;
        rho_address = rho_count;
        theta_address = theta_count;
        debug_state = READ;
        
        if (rho_count >= nrho-1)
            rho_count = fi(0, 0, 16, 0);
            if (theta_count >= ntheta-1)
                theta_count = fi(0, 0, 8, 0);
                if (k_count >= ktheta-2)
                    k_count = fi(0, 0, 8, 0);
                    current_state = CLEAR;
                else
                    k_count = fi(k_count + 1, 0, 8, 0);
                    current_state = READ;
                end
            else
                theta_count = fi(theta_count + 1, 0, 8, 0);
                current_state = READ;
            end
        else
            rho_count = fi(rho_count + 1, 0, 16, 0);
            current_state = READ;
        end
        
    case CLEAR
        mode = false;
        valid = true;
        clear = true;
        rho_address = rho_count;
        theta_address = theta_count;
        debug_state = CLEAR;
        
        if (rho_count >= nrho-1)
            rho_count = fi(0, 0, 16, 0);
            if (theta_count >= ntheta-1)
                theta_count = fi(0, 0, 8, 0);
                current_state = IDLE;
            else
                theta_count = fi(theta_count + 1, 0, 8, 0);
                current_state = CLEAR;
            end
        else
            rho_count = fi(rho_count + 1, 0, 16, 0);
            current_state = CLEAR;
        end
        
    otherwise
        mode = false;
        valid = false;
        clear = false;
        rho_address = rho_count;
        theta_address = theta_count;
        debug_state = IDLE;
        
        current_state = IDLE;
        
end

== matlab function library/RBM Circuit/RBM Controller ==
  data: sof input; mode output; rho_address output; theta_address output; eof input; ntheta input; nrho input; clear output; debug_state output
function [mode, rho_address, theta_address, clear, debug_state] = fcn(sof, eof, ntheta, nrho)

IDLE = fi(0, 0, 2, 0);
VOTE = fi(1, 0, 2, 0);
CLEAR = fi(2, 0, 2, 0);

persistent current_state;
persistent rho_count;
persistent theta_count;

if isempty(current_state)
    current_state = IDLE;
end

if isempty(rho_count)
    rho_count = fi(0, 0, 16, 0);
end

if isempty(theta_count)
    theta_count = fi(0, 0, 8, 0);
end

switch current_state
    case IDLE
        mode = false;
        clear = false;
        rho_address = rho_count;
        theta_address = theta_count;
        debug_state = IDLE;
        
        if sof
            current_state = VOTE;
        else
            current_state = IDLE;
        end
        
    case VOTE
        mode = true;
        clear = false;
        rho_address = rho_count;
        theta_address = theta_count;
        debug_state = VOTE;
        
        if eof
            current_state = CLEAR;
        else
            current_state = VOTE;
        end
        
    case CLEAR
        mode = false;
        clear = true;
        rho_address = rho_count;
        theta_address = theta_count;
        debug_state = CLEAR;
        
        if (rho_count >= nrho-1)
            rho_count = fi(0, 0, 16, 0);
            if (theta_count >= ntheta-1)
                theta_count = fi(0, 0, 8, 0);
                current_state = IDLE;
            else
                theta_count = fi(theta_count + 1, 0, 8, 0);
                current_state = CLEAR;
            end
        else
            rho_count = fi(rho_count + 1, 0, 16, 0);
            current_state = CLEAR;
        end
        
    otherwise
        mode = false;
        clear = false;
        rho_address = rho_count;
        theta_address = theta_count;
        debug_state = IDLE
        
        current_state = IDLE;
        
end
